simulink model "Marquez_No1simulink"  (R2023b)
settings: Solver=VariableStepAuto  StartTime=0.0  StopTime=20.0  RelTol=1e-3
values from neighbouring files (symbols this model uses):
  P_den = [M B k]    [Marquez_No1.m]
  P_num = [1]    [Marquez_No1.m]
settings Model: Creator=Princess  LastModifiedBy=Princess

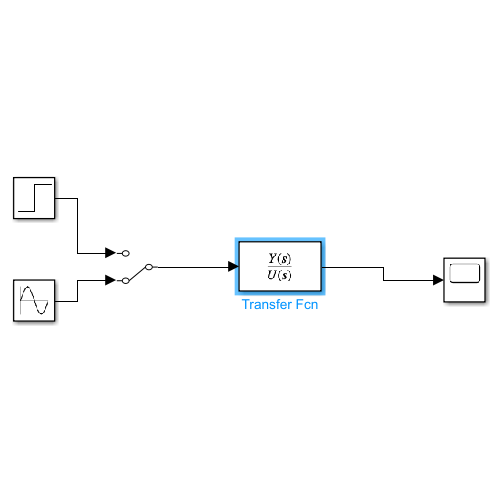
[thumbnail: Simulink's stored preview of the top-level diagram]
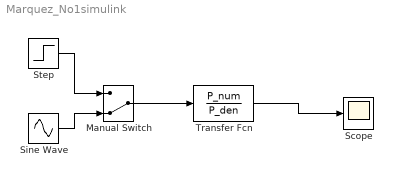
== system Marquez_No1simulink ==
  Manual Switch : ManualSwitch  CurrentSetting=0
  Scope : Scope
  Sine Wave : Sin  SampleTime=0
  Step : Step  Time=0  SampleTime=0
  Transfer Fcn : TransferFcn  Numerator=P_num  Denominator=P_den
  wires:
  Transfer Fcn/1 -> Scope/1
  Manual Switch/1 -> Transfer Fcn/1
  Step/1 -> Manual Switch/1
  Sine Wave/1 -> Manual Switch/2
